simulink model "SingleTrack"  (R2019b)
settings: Solver=ode1  StartTime=0  StopTime=250  FixedStep=1.0000000000000000e-003  RelTol=1e-3
InitFcn:
  | sampleTime = str2double(get_param(bdroot, 'FixedStep'));
undefined symbols (not defined in the file or in its folder): AccPedalPos, BrakePedalPos, BrakeSwitch, DiscIntNeverNeededParam, DYNA4, EngSpd, IgnitionSwitch, InitialGear, InitialSpeed, IntendedEngTrq, LeftIndicator, MainBrakePress, MaxGear, MDL, MinGear, RefAcc, RefLane, RefLatPos, RefPath, RefPathCurv, RefSpd, RefSpdPreview, RefSpdRetrospect, RightIndicator, SteeringWheelAng, SteeringWheelTrq, UserDefinedRefValue, vm_const
libraries: UtilitiesLibrary x31, simulink x18, WheelSystemModules x13, LongitudinalControllerModules x13, LateralControllerModules x7, AnimationBusselectorModules x5, EnvironmentModules x5, BasicEngineControlModules x5, MiscellaneousControlModules x5, Animation3Modules x4, AuxiliariesModules x4, ReducedTireModules x4
(part 29 of 32)

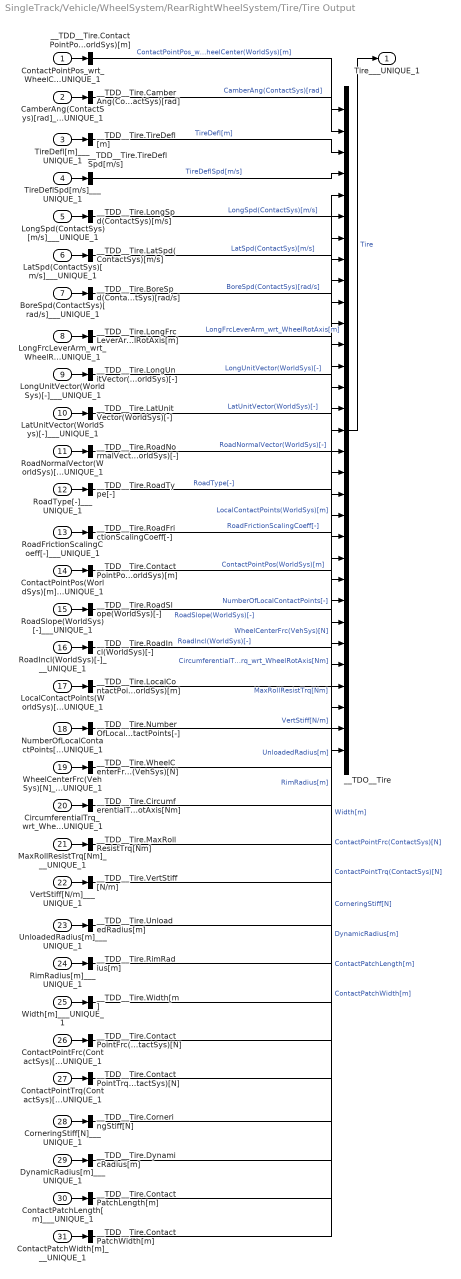
== system SingleTrack/Vehicle/WheelSystem/RearRightWheelSystem/Tire/Tire Output ==
  ContactPointPos_wrt_WheelCenter(WorldSys)[m]___UNIQUE_1 : Inport  Description=|  PortDimensions=[3]
      | <name>ContactPointPos_wrt_WheelCenter(WorldSys)[m]</name>
      | <comment></comment>
  CamberAng(ContactSys)[rad]___UNIQUE_1 : Inport  Description=|  Port=2  PortDimensions=[1]
      | <name>CamberAng(ContactSys)[rad]</name>
      | <comment></comment>
  TireDefl[m]___UNIQUE_1 : Inport  Description=|  Port=3  PortDimensions=[1]
      | <name>TireDefl[m]</name>
      | <comment></comment>
  TireDeflSpd[m/s]___UNIQUE_1 : Inport  Description=|  Port=4  PortDimensions=[1]
      | <name>TireDeflSpd[m/s]</name>
      | <comment></comment>
  LongSpd(ContactSys)[m/s]___UNIQUE_1 : Inport  Description=|  Port=5  PortDimensions=[1]
      | <name>LongSpd(ContactSys)[m/s]</name>
      | <comment></comment>
  LatSpd(ContactSys)[m/s]___UNIQUE_1 : Inport  Description=|  Port=6  PortDimensions=[1]
      | <name>LatSpd(ContactSys)[m/s]</name>
      | <comment></comment>
  BoreSpd(ContactSys)[rad/s]___UNIQUE_1 : Inport  Description=|  Port=7  PortDimensions=[1]
      | <name>BoreSpd(ContactSys)[rad/s]</name>
      | <comment></comment>
  LongFrcLeverArm_wrt_WheelRotAxis[m]___UNIQUE_1 : Inport  Description=|  Port=8  PortDimensions=[1]
      | <name>LongFrcLeverArm_wrt_WheelRotAxis[m]</name>
      | <comment></comment>
  LongUnitVector(WorldSys)[-]___UNIQUE_1 : Inport  Description=|  Port=9  PortDimensions=[3]
      | <name>LongUnitVector(WorldSys)[-]</name>
      | <comment></comment>
  LatUnitVector(WorldSys)[-]___UNIQUE_1 : Inport  Description=|  Port=10  PortDimensions=[3]
      | <name>LatUnitVector(WorldSys)[-]</name>
      | <comment></comment>
  RoadNormalVector(WorldSys)[-]___UNIQUE_1 : Inport  Description=|  Port=11  PortDimensions=[3]
      | <name>RoadNormalVector(WorldSys)[-]</name>
      | <comment></comment>
  RoadType[-]___UNIQUE_1 : Inport  Description=|  Port=12  PortDimensions=[1]
      | <name>RoadType[-]</name>
      | <comment></comment>
  RoadFrictionScalingCoeff[-]___UNIQUE_1 : Inport  Description=|  Port=13  PortDimensions=[1]
      | <name>RoadFrictionScalingCoeff[-]</name>
      | <comment></comment>
  ContactPointPos(WorldSys)[m]___UNIQUE_1 : Inport  Description=|  Port=14  PortDimensions=[3]
      | <name>ContactPointPos(WorldSys)[m]</name>
      | <comment></comment>
  RoadSlope(WorldSys)[-]___UNIQUE_1 : Inport  Description=|  Port=15  PortDimensions=[1]
      | <name>RoadSlope(WorldSys)[-]</name>
      | <comment></comment>
  RoadIncl(WorldSys)[-]___UNIQUE_1 : Inport  Description=|  Port=16  PortDimensions=[1]
      | <name>RoadIncl(WorldSys)[-]</name>
      | <comment></comment>
  LocalContactPoints(WorldSys)[m]___UNIQUE_1 : Inport  Description=|  Port=17  PortDimensions=[12]
      | <name>LocalContactPoints(WorldSys)[m]</name>
      | <comment></comment>
  NumberOfLocalContactPoints[-]___UNIQUE_1 : Inport  Description=|  Port=18  PortDimensions=[1]
      | <name>NumberOfLocalContactPoints[-]</name>
      | <comment></comment>
  WheelCenterFrc(VehSys)[N]___UNIQUE_1 : Inport  Description=|  Port=19  PortDimensions=[3]
      | <name>WheelCenterFrc(VehSys)[N]</name>
      | <comment></comment>
  CircumferentialTrq_wrt_WheelRotAxis[Nm]___UNIQUE_1 : Inport  Description=|  Port=20  PortDimensions=[1]
      | <name>CircumferentialTrq_wrt_WheelRotAxis[Nm]</name>
      | <comment></comment>
  MaxRollResistTrq[Nm]___UNIQUE_1 : Inport  Description=|  Port=21  PortDimensions=[1]
      | <name>MaxRollResistTrq[Nm]</name>
      | <comment></comment>
  VertStiff[N/m]___UNIQUE_1 : Inport  Description=|  Port=22  PortDimensions=[1]
      | <name>VertStiff[N/m]</name>
      | <comment></comment>
  UnloadedRadius[m]___UNIQUE_1 : Inport  Description=|  Port=23  PortDimensions=[1]
      | <name>UnloadedRadius[m]</name>
      | <comment></comment>
  RimRadius[m]___UNIQUE_1 : Inport  Description=|  Port=24  PortDimensions=[1]
      | <name>RimRadius[m]</name>
      | <comment></comment>
  Width[m]___UNIQUE_1 : Inport  Description=|  Port=25  PortDimensions=[1]
      | <name>Width[m]</name>
      | <comment></comment>
  ContactPointFrc(ContactSys)[N]___UNIQUE_1 : Inport  Description=|  Port=26  PortDimensions=[3]
      | <name>ContactPointFrc(ContactSys)[N]</name>
      | <comment></comment>
  ContactPointTrq(ContactSys)[N]___UNIQUE_1 : Inport  Description=|  Port=27  PortDimensions=[3]
      | <name>ContactPointTrq(ContactSys)[N]</name>
      | <comment></comment>
  CorneringStiff[N]___UNIQUE_1 : Inport  Description=|  Port=28  PortDimensions=[1]
      | <name>CorneringStiff[N]</name>
      | <comment></comment>
  DynamicRadius[m]___UNIQUE_1 : Inport  Description=|  Port=29  PortDimensions=[1]
      | <name>DynamicRadius[m]</name>
      | <comment></comment>
  ContactPatchLength[m]___UNIQUE_1 : Inport  Description=|  Port=30  PortDimensions=[1]
      | <name>ContactPatchLength[m]</name>
      | <comment></comment>
  ContactPatchWidth[m]___UNIQUE_1 : Inport  Description=|  Port=31  PortDimensions=[1]
      | <name>ContactPatchWidth[m]</name>
      | <comment></comment>
  __TDD__Tire.BoreSpd(ContactSys)[rad/s] : Demux  Outputs=[1]
  __TDD__Tire.CamberAng(ContactSys)[rad] : Demux  Outputs=[1]
  __TDD__Tire.CircumferentialTrq_wrt_WheelRotAxis[Nm] : Demux  Outputs=[1]
  __TDD__Tire.ContactPatchLength[m] : Demux  Outputs=[1]
  __TDD__Tire.ContactPatchWidth[m] : Demux  Outputs=[1]
  __TDD__Tire.ContactPointFrc(ContactSys)[N] : Demux  Outputs=[3]
  __TDD__Tire.ContactPointPos(WorldSys)[m] : Demux  Outputs=[3]
  __TDD__Tire.ContactPointPos_wrt_WheelCenter(WorldSys)[m] : Demux  Outputs=[3]
  __TDD__Tire.ContactPointTrq(ContactSys)[N] : Demux  Outputs=[3]
  __TDD__Tire.CorneringStiff[N] : Demux  Outputs=[1]
  __TDD__Tire.DynamicRadius[m] : Demux  Outputs=[1]
  __TDD__Tire.LatSpd(ContactSys)[m/s] : Demux  Outputs=[1]
  __TDD__Tire.LatUnitVector(WorldSys)[-] : Demux  Outputs=[3]
  __TDD__Tire.LocalContactPoints(WorldSys)[m] : Demux  Outputs=[12]
  __TDD__Tire.LongFrcLeverArm_wrt_WheelRotAxis[m] : Demux  Outputs=[1]
  __TDD__Tire.LongSpd(ContactSys)[m/s] : Demux  Outputs=[1]
  __TDD__Tire.LongUnitVector(WorldSys)[-] : Demux  Outputs=[3]
  __TDD__Tire.MaxRollResistTrq[Nm] : Demux  Outputs=[1]
  __TDD__Tire.NumberOfLocalContactPoints[-] : Demux  Outputs=[1]
  __TDD__Tire.RimRadius[m] : Demux  Outputs=[1]
  __TDD__Tire.RoadFrictionScalingCoeff[-] : Demux  Outputs=[1]
  __TDD__Tire.RoadIncl(WorldSys)[-] : Demux  Outputs=[1]
  __TDD__Tire.RoadNormalVector(WorldSys)[-] : Demux  Outputs=[3]
  __TDD__Tire.RoadSlope(WorldSys)[-] : Demux  Outputs=[1]
  __TDD__Tire.RoadType[-] : Demux  Outputs=[1]
  __TDD__Tire.TireDeflSpd[m/s] : Demux  Outputs=[1]
  __TDD__Tire.TireDefl[m] : Demux  Outputs=[1]
  __TDD__Tire.UnloadedRadius[m] : Demux  Outputs=[1]
  __TDD__Tire.VertStiff[N/m] : Demux  Outputs=[1]
  __TDD__Tire.WheelCenterFrc(VehSys)[N] : Demux  Outputs=[3]
  __TDD__Tire.Width[m] : Demux  Outputs=[1]
  __TDO__Tire : BusCreator  Inputs=31
  Tire___UNIQUE_1 : Outport  Description=|  PortDimensions=[58]  VectorParamsAs1DForOutWhenUnconnected=off
      | <name>ContactPointPos_wrt_WheelCenter(WorldSys)[m]</name>
      | <comment></comment>
  wires:
  __TDO__Tire/1 -> Tire___UNIQUE_1/1  "Tire"
  __TDD__Tire.ContactPatchWidth[m]/1 -> __TDO__Tire/31  "ContactPatchWidth[m]"
  ContactPatchWidth[m]___UNIQUE_1/1 -> __TDD__Tire.ContactPatchWidth[m]/1
  __TDD__Tire.ContactPatchLength[m]/1 -> __TDO__Tire/30  "ContactPatchLength[m]"
  ContactPatchLength[m]___UNIQUE_1/1 -> __TDD__Tire.ContactPatchLength[m]/1
  __TDD__Tire.DynamicRadius[m]/1 -> __TDO__Tire/29  "DynamicRadius[m]"
  DynamicRadius[m]___UNIQUE_1/1 -> __TDD__Tire.DynamicRadius[m]/1
  __TDD__Tire.CorneringStiff[N]/1 -> __TDO__Tire/28  "CorneringStiff[N]"
  CorneringStiff[N]___UNIQUE_1/1 -> __TDD__Tire.CorneringStiff[N]/1
  __TDD__Tire.ContactPointTrq(ContactSys)[N]/1 -> __TDO__Tire/27  "ContactPointTrq(ContactSys)[N]"
  ContactPointTrq(ContactSys)[N]___UNIQUE_1/1 -> __TDD__Tire.ContactPointTrq(ContactSys)[N]/1
  __TDD__Tire.ContactPointFrc(ContactSys)[N]/1 -> __TDO__Tire/26  "ContactPointFrc(ContactSys)[N]"
  ContactPointFrc(ContactSys)[N]___UNIQUE_1/1 -> __TDD__Tire.ContactPointFrc(ContactSys)[N]/1
  __TDD__Tire.Width[m]/1 -> __TDO__Tire/25  "Width[m]"
  Width[m]___UNIQUE_1/1 -> __TDD__Tire.Width[m]/1
  __TDD__Tire.RimRadius[m]/1 -> __TDO__Tire/24  "RimRadius[m]"
  RimRadius[m]___UNIQUE_1/1 -> __TDD__Tire.RimRadius[m]/1
  __TDD__Tire.UnloadedRadius[m]/1 -> __TDO__Tire/23  "UnloadedRadius[m]"
  UnloadedRadius[m]___UNIQUE_1/1 -> __TDD__Tire.UnloadedRadius[m]/1
  __TDD__Tire.VertStiff[N/m]/1 -> __TDO__Tire/22  "VertStiff[N/m]"
  VertStiff[N/m]___UNIQUE_1/1 -> __TDD__Tire.VertStiff[N/m]/1
  __TDD__Tire.MaxRollResistTrq[Nm]/1 -> __TDO__Tire/21  "MaxRollResistTrq[Nm]"
  MaxRollResistTrq[Nm]___UNIQUE_1/1 -> __TDD__Tire.MaxRollResistTrq[Nm]/1
  __TDD__Tire.CircumferentialTrq_wrt_WheelRotAxis[Nm]/1 -> __TDO__Tire/20  "CircumferentialTrq_wrt_WheelRotAxis[Nm]"
  CircumferentialTrq_wrt_WheelRotAxis[Nm]___UNIQUE_1/1 -> __TDD__Tire.CircumferentialTrq_wrt_WheelRotAxis[Nm]/1
  __TDD__Tire.WheelCenterFrc(VehSys)[N]/1 -> __TDO__Tire/19  "WheelCenterFrc(VehSys)[N]"
  WheelCenterFrc(VehSys)[N]___UNIQUE_1/1 -> __TDD__Tire.WheelCenterFrc(VehSys)[N]/1
  __TDD__Tire.NumberOfLocalContactPoints[-]/1 -> __TDO__Tire/18  "NumberOfLocalContactPoints[-]"
  NumberOfLocalContactPoints[-]___UNIQUE_1/1 -> __TDD__Tire.NumberOfLocalContactPoints[-]/1
  __TDD__Tire.LocalContactPoints(WorldSys)[m]/1 -> __TDO__Tire/17  "LocalContactPoints(WorldSys)[m]"
  LocalContactPoints(WorldSys)[m]___UNIQUE_1/1 -> __TDD__Tire.LocalContactPoints(WorldSys)[m]/1
  __TDD__Tire.RoadIncl(WorldSys)[-]/1 -> __TDO__Tire/16  "RoadIncl(WorldSys)[-]"
  RoadIncl(WorldSys)[-]___UNIQUE_1/1 -> __TDD__Tire.RoadIncl(WorldSys)[-]/1
  __TDD__Tire.RoadSlope(WorldSys)[-]/1 -> __TDO__Tire/15  "RoadSlope(WorldSys)[-]"
  RoadSlope(WorldSys)[-]___UNIQUE_1/1 -> __TDD__Tire.RoadSlope(WorldSys)[-]/1
  __TDD__Tire.ContactPointPos(WorldSys)[m]/1 -> __TDO__Tire/14  "ContactPointPos(WorldSys)[m]"
  ContactPointPos(WorldSys)[m]___UNIQUE_1/1 -> __TDD__Tire.ContactPointPos(WorldSys)[m]/1
  __TDD__Tire.RoadFrictionScalingCoeff[-]/1 -> __TDO__Tire/13  "RoadFrictionScalingCoeff[-]"
  RoadFrictionScalingCoeff[-]___UNIQUE_1/1 -> __TDD__Tire.RoadFrictionScalingCoeff[-]/1
  __TDD__Tire.RoadType[-]/1 -> __TDO__Tire/12  "RoadType[-]"
  RoadType[-]___UNIQUE_1/1 -> __TDD__Tire.RoadType[-]/1
  __TDD__Tire.RoadNormalVector(WorldSys)[-]/1 -> __TDO__Tire/11  "RoadNormalVector(WorldSys)[-]"
  RoadNormalVector(WorldSys)[-]___UNIQUE_1/1 -> __TDD__Tire.RoadNormalVector(WorldSys)[-]/1
  __TDD__Tire.LatUnitVector(WorldSys)[-]/1 -> __TDO__Tire/10  "LatUnitVector(WorldSys)[-]"
  LatUnitVector(WorldSys)[-]___UNIQUE_1/1 -> __TDD__Tire.LatUnitVector(WorldSys)[-]/1
  __TDD__Tire.LongUnitVector(WorldSys)[-]/1 -> __TDO__Tire/9  "LongUnitVector(WorldSys)[-]"
  LongUnitVector(WorldSys)[-]___UNIQUE_1/1 -> __TDD__Tire.LongUnitVector(WorldSys)[-]/1
  __TDD__Tire.LongFrcLeverArm_wrt_WheelRotAxis[m]/1 -> __TDO__Tire/8  "LongFrcLeverArm_wrt_WheelRotAxis[m]"
  LongFrcLeverArm_wrt_WheelRotAxis[m]___UNIQUE_1/1 -> __TDD__Tire.LongFrcLeverArm_wrt_WheelRotAxis[m]/1
  __TDD__Tire.BoreSpd(ContactSys)[rad/s]/1 -> __TDO__Tire/7  "BoreSpd(ContactSys)[rad/s]"
  BoreSpd(ContactSys)[rad/s]___UNIQUE_1/1 -> __TDD__Tire.BoreSpd(ContactSys)[rad/s]/1
  __TDD__Tire.LatSpd(ContactSys)[m/s]/1 -> __TDO__Tire/6  "LatSpd(ContactSys)[m/s]"
  LatSpd(ContactSys)[m/s]___UNIQUE_1/1 -> __TDD__Tire.LatSpd(ContactSys)[m/s]/1
  __TDD__Tire.LongSpd(ContactSys)[m/s]/1 -> __TDO__Tire/5  "LongSpd(ContactSys)[m/s]"
  LongSpd(ContactSys)[m/s]___UNIQUE_1/1 -> __TDD__Tire.LongSpd(ContactSys)[m/s]/1
  __TDD__Tire.TireDeflSpd[m/s]/1 -> __TDO__Tire/4  "TireDeflSpd[m/s]"
  TireDeflSpd[m/s]___UNIQUE_1/1 -> __TDD__Tire.TireDeflSpd[m/s]/1
  __TDD__Tire.TireDefl[m]/1 -> __TDO__Tire/3  "TireDefl[m]"
  TireDefl[m]___UNIQUE_1/1 -> __TDD__Tire.TireDefl[m]/1
  __TDD__Tire.CamberAng(ContactSys)[rad]/1 -> __TDO__Tire/2  "CamberAng(ContactSys)[rad]"
  CamberAng(ContactSys)[rad]___UNIQUE_1/1 -> __TDD__Tire.CamberAng(ContactSys)[rad]/1
  __TDD__Tire.ContactPointPos_wrt_WheelCenter(WorldSys)[m]/1 -> __TDO__Tire/1  "ContactPointPos_wrt_WheelCenter(WorldSys)[m]"
  ContactPointPos_wrt_WheelCenter(WorldSys)[m]___UNIQUE_1/1 -> __TDD__Tire.ContactPointPos_wrt_WheelCenter(WorldSys)[m]/1

== system SingleTrack/Vehicle/WheelSystem/WheelSystemOutputs/WheelRear2//3Output/WheelSystemOutput ==
  __SEL__WheelSystem.InnerTire.ContactPointFrc(ContactSys)[N] : Selector  InputPortWidth=1  IndexOptions=Index vector (dialog)  Indices=ones(3, 1)  OutputSizes=1
  __SEL__WheelSystem.InnerTire.ContactPointPos(WorldSys)[m] : Selector  InputPortWidth=1  IndexOptions=Index vector (dialog)  Indices=ones(3, 1)  OutputSizes=1
  __SEL__WheelSystem.Tire.ContactPointFrc(ContactSys)[N] : Selector  InputPortWidth=1  IndexOptions=Index vector (dialog)  Indices=ones(3, 1)  OutputSizes=1
  __SEL__WheelSystem.Tire.ContactPointPos(WorldSys)[m] : Selector  InputPortWidth=1  IndexOptions=Index vector (dialog)  Indices=ones(3, 1)  OutputSizes=1
  __SRC__WheelSystem.InnerTire.ContactPointFrc(ContactSys)[N] : Constant  Value=0.0  OutDataTypeStr=Inherit: Inherit via back propagation
  __SRC__WheelSystem.InnerTire.ContactPointPos(WorldSys)[m] : Constant  Value=0.0  OutDataTypeStr=Inherit: Inherit via back propagation
  __SRC__WheelSystem.InnerTire.MaxRollResistTrq[Nm] : Constant  Value=0.0  OutDataTypeStr=Inherit: Inherit via back propagation
  __SRC__WheelSystem.Tire.ContactPointFrc(ContactSys)[N] : Constant  Value=0.0  OutDataTypeStr=Inherit: Inherit via back propagation
  __SRC__WheelSystem.Tire.ContactPointPos(WorldSys)[m] : Constant  Value=0.0  OutDataTypeStr=Inherit: Inherit via back propagation
  __SRC__WheelSystem.Tire.MaxRollResistTrq[Nm] : Constant  Value=0.0  OutDataTypeStr=Inherit: Inherit via back propagation
  __SRC__WheelSystem.Wheel.RotAcc[rad/s**2] : Constant  Value=0.0  OutDataTypeStr=Inherit: Inherit via back propagation
  __SRC__WheelSystem.Wheel.RotAng[rad] : Constant  Value=0.0  OutDataTypeStr=Inherit: Inherit via back propagation
  __SRC__WheelSystem.Wheel.RotAxisInrt[kg*m**2] : Constant  Value=0.0  OutDataTypeStr=Inherit: Inherit via back propagation
  __SRC__WheelSystem.Wheel.RotSpd[rad/s] : Constant  Value=0.0  OutDataTypeStr=Inherit: Inherit via back propagation
  __TDO__WheelSystem : BusCreator  Inputs=3
  __TDO__WheelSystem.InnerTire : BusCreator  Inputs=3
  __TDO__WheelSystem.Tire : BusCreator  Inputs=3
  __TDO__WheelSystem.Wheel : BusCreator  Inputs=4
  WheelSystem___UNIQUE_1 : Outport  Description=|  PortDimensions=[18]  VectorParamsAs1DForOutWhenUnconnected=off
      | <name></name>
      | <comment></comment>
  wires:
  __TDO__WheelSystem/1 -> WheelSystem___UNIQUE_1/1  "WheelSystem"
  __SEL__WheelSystem.InnerTire.ContactPointFrc(ContactSys)[N]/1 -> __TDO__WheelSystem.InnerTire/3  "ContactPointFrc(ContactSys)[N]"
  __SEL__WheelSystem.InnerTire.ContactPointPos(WorldSys)[m]/1 -> __TDO__WheelSystem.InnerTire/2  "ContactPointPos(WorldSys)[m]"
  __SEL__WheelSystem.Tire.ContactPointFrc(ContactSys)[N]/1 -> __TDO__WheelSystem.Tire/3  "ContactPointFrc(ContactSys)[N]"
  __SEL__WheelSystem.Tire.ContactPointPos(WorldSys)[m]/1 -> __TDO__WheelSystem.Tire/2  "ContactPointPos(WorldSys)[m]"
  __SRC__WheelSystem.Wheel.RotAng[rad]/1 -> __TDO__WheelSystem.Wheel/4  "RotAng[rad]"
  __TDO__WheelSystem.InnerTire/1 -> __TDO__WheelSystem/3  "InnerTire"
  __SRC__WheelSystem.InnerTire.MaxRollResistTrq[Nm]/1 -> __TDO__WheelSystem.InnerTire/1  "MaxRollResistTrq[Nm]"
  __TDO__WheelSystem.Tire/1 -> __TDO__WheelSystem/2  "Tire"
  __SRC__WheelSystem.Tire.MaxRollResistTrq[Nm]/1 -> __TDO__WheelSystem.Tire/1  "MaxRollResistTrq[Nm]"
  __SRC__WheelSystem.Wheel.RotAxisInrt[kg*m**2]/1 -> __TDO__WheelSystem.Wheel/3  "RotAxisInrt[kg*m**2]"
  __SRC__WheelSystem.Wheel.RotAcc[rad/s**2]/1 -> __TDO__WheelSystem.Wheel/2  "RotAcc[rad/s**2]"
  __TDO__WheelSystem.Wheel/1 -> __TDO__WheelSystem/1  "Wheel"
  __SRC__WheelSystem.Wheel.RotSpd[rad/s]/1 -> __TDO__WheelSystem.Wheel/1  "RotSpd[rad/s]"
  __SRC__WheelSystem.InnerTire.ContactPointFrc(ContactSys)[N]/1 -> __SEL__WheelSystem.InnerTire.ContactPointFrc(ContactSys)[N]/1
  __SRC__WheelSystem.InnerTire.ContactPointPos(WorldSys)[m]/1 -> __SEL__WheelSystem.InnerTire.ContactPointPos(WorldSys)[m]/1
  __SRC__WheelSystem.Tire.ContactPointFrc(ContactSys)[N]/1 -> __SEL__WheelSystem.Tire.ContactPointFrc(ContactSys)[N]/1
  __SRC__WheelSystem.Tire.ContactPointPos(WorldSys)[m]/1 -> __SEL__WheelSystem.Tire.ContactPointPos(WorldSys)[m]/1

== system SingleTrack/VehicleControl/LateralControl/Disabled LateralControl/ControlSystems/Control Systems Parameters ==
  CurvatureControl : Subsystem
      settings: CopyFcn=DYNA4.Internal.ModelCallbacks.Modules.UpdateMaskParameters(gcb);  NameChangeFcn=DYNA4.Internal.ModelCallbacks.Modules.UpdateMaskParameters(gcb);
  PathControl : Subsystem
      settings: CopyFcn=DYNA4.Internal.ModelCallbacks.Modules.UpdateMaskParameters(gcb);  NameChangeFcn=DYNA4.Internal.ModelCallbacks.Modules.UpdateMaskParameters(gcb);

== system SingleTrack/VehicleControl/LateralControl/Disabled LateralControl/ControlSystems/DynaSystemInfo ==

== system SingleTrack/VehicleControl/LateralControl/Disabled LateralControl/ControlSystems/Lateral Controller ==
  User-Defined Control : Subsystem  TreatAsAtomicUnit=on

== system SingleTrack/VehicleControl/LateralControl/Disabled LateralControl/ControlSystems/LateralControlOutput ==
  __SRC__LateralControl.LateralPhase : Constant  Value=0.0  OutDataTypeStr=Inherit: Inherit via back propagation
  __SRC__LateralControl.LeftIndicator : Constant  Value=0.0  OutDataTypeStr=Inherit: Inherit via back propagation
  __SRC__LateralControl.RightIndicator : Constant  Value=0.0  OutDataTypeStr=Inherit: Inherit via back propagation
  __SRC__LateralControl.SteeringWheelAng : Constant  Value=0.0  OutDataTypeStr=Inherit: Inherit via back propagation
  __SRC__LateralControl.SteeringWheelInputSwitch : Constant  Value=0.0  OutDataTypeStr=Inherit: Inherit via back propagation
  __SRC__LateralControl.SteeringWheelTrq : Constant  Value=0.0  OutDataTypeStr=Inherit: Inherit via back propagation
  __SRC__LateralControl.UserDefined1 : Constant  Value=0.0  OutDataTypeStr=Inherit: Inherit via back propagation
  __SRC__LateralControl.UserDefined2 : Constant  Value=0.0  OutDataTypeStr=Inherit: Inherit via back propagation
  __SRC__LateralControl.UserDefinedRefValue : Constant  Value=0.0  OutDataTypeStr=Inherit: Inherit via back propagation
  __TDO__LateralControl : BusCreator  Inputs=9
  LateralControl___UNIQUE_1 : Outport  Description=|  PortDimensions=[9]  VectorParamsAs1DForOutWhenUnconnected=off
      | <name>SteeringWheelAng</name>
      | <comment>Steering wheel angle</comment>
  wires:
  __TDO__LateralControl/1 -> LateralControl___UNIQUE_1/1  "LateralControl"
  __SRC__LateralControl.UserDefined2/1 -> __TDO__LateralControl/9  "UserDefined2[-]"
  __SRC__LateralControl.UserDefined1/1 -> __TDO__LateralControl/8  "UserDefined1[-]"
  __SRC__LateralControl.LateralPhase/1 -> __TDO__LateralControl/7  "LateralPhase[-]"
  __SRC__LateralControl.RightIndicator/1 -> __TDO__LateralControl/6  "RightIndicator[0;1]"
  __SRC__LateralControl.LeftIndicator/1 -> __TDO__LateralControl/5  "LeftIndicator[0;1]"
  __SRC__LateralControl.UserDefinedRefValue/1 -> __TDO__LateralControl/4  "UserDefinedRefValue[-]"
  __SRC__LateralControl.SteeringWheelInputSwitch/1 -> __TDO__LateralControl/3  "SteeringWheelInputSwitch[-]"
  __SRC__LateralControl.SteeringWheelTrq/1 -> __TDO__LateralControl/2  "SteeringWheelTrq[Nm]"
  __SRC__LateralControl.SteeringWheelAng/1 -> __TDO__LateralControl/1  "SteeringWheelAng[rad]"

== system SingleTrack/VehicleControl/LateralControl/Disabled LateralControl/ControlSystemsPreprocessor/Maneuver ==
  DynaModuleInfo : Subsystem  Tag=DynaModuleInfo
      mask init:
      | data = get_param(gcb, 'UserData');
      mask Display: disp(['Type = ', data.type, '\nName = ', char(data.name)]);

== system SingleTrack/VehicleControl/LateralControl/Enabled LateralControl/ControlSystems/Control Systems Parameters ==
  note: TASK_LAT_STEERING_WHEEL_ANG = 1;
      | 	TASK_LAT_STEERING_WHEEL_TORQUE = 2;
      | 	TASK_LAT_PATH_CONTROL = 3;
      | 	TASK_LAT_CURVATURE_CONTROL = 4;
      | 	TASK_LAT_USER_DEFINED = 5;
  TaskIdentifier : Inport
  CtrlSystemsAbscissae : Inport  Port=2
  Bus Selector : BusSelector  OutputSignals=Task
  CurvatureControl : LateralControllerModules/DataContainerCurvatureControl  DATA_NODE=MDL.VehicleControl.LateralControl.ControlSystems.CurvatureControl  PreviewDist=MDL.VehicleControl.LateralControl.ControlSystems.CurvatureControl.PreviewDist  PreviewTime=MDL.VehicleControl.LateralControl.ControlSystems.CurvatureControl.PreviewTime  TargetAimDist=MDL.VehicleControl.LateralControl.ControlSystems.CurvatureControl.TargetAimDist  MaxLeftSteeringRate=MDL.VehicleControl.LateralControl.ControlSystems.CurvatureControl.MaxLeftSteeringRate  MaxRightSteeringRate=MDL.VehicleControl.LateralControl.ControlSystems.CurvatureControl.MaxRightSteeringRate  SteeringAngSmoothTimeConst=MDL.VehicleControl.LateralControl.ControlSystems.CurvatureControl.SteeringAngSmoothTimeConst  LatCtrlGain=MDL.VehicleControl.LateralControl.ControlSystems.CurvatureControl.LatCtrlGain  ControllerDeviationScaling=MDL.VehicleControl.LateralControl.ControlSystems.CurvatureControl.ControllerDeviationScaling  FrontAxleLatStiff=MDL.VehicleControl.LateralControl.ControlSystems.CurvatureControl.FrontAxleLatStiff  RearAxleLatStiff=MDL.VehicleControl.LateralControl.ControlSystems.CurvatureControl.RearAxleLatStiff  RearTiresLatFrcSmoothTimeConst=MDL.VehicleControl.LateralControl.ControlSystems.CurvatureControl.RearTiresLatFrcSmoothTimeConst  RearTiresLatFrcSwitch=MDL.VehicleControl.LateralControl.ControlSystems.CurvatureControl.RearTiresLatFrcSwitch  RearTiresLatFrcScaling=MDL.VehicleControl.LateralControl.ControlSystems.CurvatureControl.RearTiresLatFrcScaling  SmoothingInterval=MDL.VehicleControl.LateralControl.ControlSystems.CurvatureControl.SmoothingInterval  Preview=MDL.VehicleControl.LateralControl.ControlSystems.CurvatureControl.Preview  DrivingSkill=MDL.VehicleControl.LateralControl.ControlSystems.CurvatureControl.DrivingSkill  Smoothness=MDL.VehicleControl.LateralControl.ControlSystems.CurvatureControl.Smoothness
  Merge : Merge
  PathControl : LateralControllerModules/DataContainerPathControl  DATA_NODE=MDL.VehicleControl.LateralControl.ControlSystems.PathControl  PreviewDist=MDL.VehicleControl.LateralControl.ControlSystems.PathControl.PreviewDist  PreviewTime=MDL.VehicleControl.LateralControl.ControlSystems.PathControl.PreviewTime  TargetAimDist=MDL.VehicleControl.LateralControl.ControlSystems.PathControl.TargetAimDist  MaxLeftSteeringRate=MDL.VehicleControl.LateralControl.ControlSystems.PathControl.MaxLeftSteeringRate  MaxRightSteeringRate=MDL.VehicleControl.LateralControl.ControlSystems.PathControl.MaxRightSteeringRate  SteeringAngSmoothTimeConst=MDL.VehicleControl.LateralControl.ControlSystems.PathControl.SteeringAngSmoothTimeConst  LatCtrlGain=MDL.VehicleControl.LateralControl.ControlSystems.PathControl.LatCtrlGain  ControllerDeviationScaling=MDL.VehicleControl.LateralControl.ControlSystems.PathControl.ControllerDeviationScaling  FrontAxleLatStiff=MDL.VehicleControl.LateralControl.ControlSystems.PathControl.FrontAxleLatStiff  RearAxleLatStiff=MDL.VehicleControl.LateralControl.ControlSystems.PathControl.RearAxleLatStiff  RearTiresLatFrcSmoothTimeConst=MDL.VehicleControl.LateralControl.ControlSystems.PathControl.RearTiresLatFrcSmoothTimeConst  RearTiresLatFrcSwitch=MDL.VehicleControl.LateralControl.ControlSystems.PathControl.RearTiresLatFrcSwitch  RearTiresLatFrcScaling=MDL.VehicleControl.LateralControl.ControlSystems.PathControl.RearTiresLatFrcScaling  LaneChangeDurationTime=MDL.VehicleControl.LateralControl.ControlSystems.PathControl.LaneChangeDurationTime  LaneChangeDurationDist=MDL.VehicleControl.LateralControl.ControlSystems.PathControl.LaneChangeDurationDist  SmoothingInterval=MDL.VehicleControl.LateralControl.ControlSystems.PathControl.SmoothingInterval  Preview=MDL.VehicleControl.LateralControl.ControlSystems.PathControl.Preview  DrivingSkill=MDL.VehicleControl.LateralControl.ControlSystems.PathControl.DrivingSkill  Smoothness=MDL.VehicleControl.LateralControl.ControlSystems.PathControl.Smoothness
  Switch Case : SwitchCase  CaseConditions={vm_const('TASK_LAT_PATH_CONTROL'), vm_const('TASK_LAT_CURVATURE_CONTROL')}  ShowDefaultCase=off
  ControllerParameters : Outport  VectorParamsAs1DForOutWhenUnconnected=off
  wires:
  Switch Case/2 -> CurvatureControl/Action
  Switch Case/1 -> PathControl/Action
  CtrlSystemsAbscissae/1 -> CurvatureControl/1, PathControl/1
  Merge/1 -> ControllerParameters/1
  CurvatureControl/1 -> Merge/2
  PathControl/1 -> Merge/1
  TaskIdentifier/1 -> Bus Selector/1
  Bus Selector/1 -> Switch Case/1  "<Task>"

== system SingleTrack/VehicleControl/LateralControl/Enabled LateralControl/ControlSystems/DynaSystemInfo ==

== system SingleTrack/VehicleControl/LateralControl/Enabled LateralControl/ControlSystems/Lateral Controller ==
  note: TASK_LAT_STEERING_WHEEL_ANG = 1;
      | 	TASK_LAT_STEERING_WHEEL_TORQUE = 2;
      | 	TASK_LAT_PATH_CONTROL = 3;
      | 	TASK_LAT_CURVATURE_CONTROL = 4;
      | 	TASK_LAT_USER_DEFINED = 5;
  TaskIdentifiers : Inport
  SourceIdentifiers : Inport  Port=2
  ControlInputs : Inport  Port=3
  ControllerParameters : Inport  Port=4
  VehicleInfo : Inport  Port=5
  Bus Selector : BusSelector  OutputSignals=Task,Subtask
  Initialization : Subsystem
  Merge : Merge  Inputs=5
  Path and Curvature Control : Subsystem  TreatAsAtomicUnit=on
  Steering Wheel Angle Input : Subsystem  TreatAsAtomicUnit=on
  Steering Wheel Torque Input : Subsystem  TreatAsAtomicUnit=on
  Switch Case : SwitchCase  CaseConditions={vm_const('TASK_LAT_STEERING_WHEEL_ANG'), vm_const('TASK_LAT_STEERING_WHEEL_TORQUE'), [vm_const('TASK_LAT_PATH_CONTROL'),vm_const('TASK_LAT_CURVATURE_CONTROL')], vm_const('TASK_LAT_USER_DEFINED')}
  User-Defined Control : Subsystem  TreatAsAtomicUnit=on
  SteeringWheelDemands : Outport  VectorParamsAs1DForOutWhenUnconnected=off
  UserDefinedRefValue[-] : Outport  Port=2  PortDimensions=1  VectorParamsAs1DForOutWhenUnconnected=off
  wires:
  Steering Wheel Torque Input/1(SteeringWheelDemands) -> Merge/2
  Switch Case/2 -> Steering Wheel Torque Input/Action
  User-Defined Control/1(SteeringWheelDemands) -> Merge/4
  Path and Curvature Control/1(SteeringWheelDemands) -> Merge/3
  Initialization/1(SteeringWheelDemands) -> Merge/5
  Switch Case/3 -> Path and Curvature Control/Action
  Switch Case/4 -> User-Defined Control/Action
  Switch Case/1 -> Steering Wheel Angle Input/Action
  Switch Case/5 -> Initialization/Action
  User-Defined Control/2(UserDefinedRefValue[-]) -> UserDefinedRefValue[-]/1
  SourceIdentifiers/1 -> User-Defined Control/3(SourceIdentifiers)
  ControlInputs/1 -> Steering Wheel Angle Input/1(ControlInputs), Steering Wheel Torque Input/1(ControlInputs), Path and Curvature Control/1(ControlInputs), User-Defined Control/1(ControlInputs)
  ControllerParameters/1 -> Path and Curvature Control/2(ControllerParameters)
  VehicleInfo/1 -> Path and Curvature Control/3(VehicleInfo), User-Defined Control/2(VehicleInfo), Steering Wheel Angle Input/2(VehicleInfo), Steering Wheel Torque Input/2(VehicleInfo)
  Merge/1 -> SteeringWheelDemands/1
  Steering Wheel Angle Input/1(SteeringWheelDemands) -> Merge/1
  TaskIdentifiers/1 -> Bus Selector/1
  Bus Selector/1 -> Switch Case/1  "<Task>"
  Bus Selector/2 -> User-Defined Control/4(SubtaskIdentifiers)  "<Subtask>"

== system SingleTrack/VehicleControl/LateralControl/Enabled LateralControl/ControlSystems/LateralControlOutput ==
  SteeringWheelAng[rad]___UNIQUE_1 : Inport  Description=|  PortDimensions=[1]
      | <name>SteeringWheelAng[rad]</name>
      | <comment>Steering wheel angle</comment>
  SteeringWheelTrq[Nm]___UNIQUE_1 : Inport  Description=|  Port=2  PortDimensions=[1]
      | <name>SteeringWheelTrq[Nm]</name>
      | <comment>Steering wheel torque</comment>
  SteeringWheelInputSwitch[-]___UNIQUE_1 : Inport  Description=|  Port=3  PortDimensions=[1]
      | <name>SteeringWheelInputSwitch[-]</name>
      | <comment>Steering wheel input switch (0: angle, 1: torque)</comment>
  UserDefinedRefValue[-]___UNIQUE_1 : Inport  Description=|  Port=4  PortDimensions=[1]
      | <name>UserDefinedRefValue[-]</name>
      | <comment>User-defined reference value</comment>
  LeftIndicator[0;1]___UNIQUE_1 : Inport  Description=|  Port=5  PortDimensions=[1]
      | <name>LeftIndicator[0;1]</name>
      | <comment>Left indicator state</comment>
  RightIndicator[0;1]___UNIQUE_1 : Inport  Description=|  Port=6  PortDimensions=[1]
      | <name>RightIndicator[0;1]</name>
      | <comment>Right indicator state</comment>
  LateralPhase[-]___UNIQUE_1 : Inport  Description=|  Port=7  PortDimensions=[1]
      | <name>LateralPhase[-]</name>
      | <comment>Lateral phase number</comment>
  UserDefined1[-]___UNIQUE_1 : Inport  Description=|  Port=8  PortDimensions=[1]
      | <name>UserDefined.UserDefined1[-]</name>
      | <comment>User-defined additional input 1 (can be edited by the user)</comment>
  UserDefined2[-]___UNIQUE_1 : Inport  Description=|  Port=9  PortDimensions=[1]
      | <name>UserDefined.UserDefined2[-]</name>
      | <comment>User-defined additional input 2 (can be edited by the user)</comment>
  __TDD__LateralControl.LateralPhase[-] : Demux  Outputs=[1]
  __TDD__LateralControl.LeftIndicator[0;1] : Demux  Outputs=[1]
  __TDD__LateralControl.RightIndicator[0;1] : Demux  Outputs=[1]
  __TDD__LateralControl.SteeringWheelAng[rad] : Demux  Outputs=[1]
  __TDD__LateralControl.SteeringWheelInputSwitch[-] : Demux  Outputs=[1]
  __TDD__LateralControl.SteeringWheelTrq[Nm] : Demux  Outputs=[1]
  __TDD__LateralControl.UserDefined1[-] : Demux  Outputs=[1]
  __TDD__LateralControl.UserDefined2[-] : Demux  Outputs=[1]
  __TDD__LateralControl.UserDefinedRefValue[-] : Demux  Outputs=[1]
  __TDO__LateralControl : BusCreator  Inputs=9
  LateralControl___UNIQUE_1 : Outport  Description=|  PortDimensions=[9]  VectorParamsAs1DForOutWhenUnconnected=off
      | <name>SteeringWheelAng[rad]</name>
      | <comment>Steering wheel angle</comment>
  wires:
  __TDO__LateralControl/1 -> LateralControl___UNIQUE_1/1  "LateralControl"
  __TDD__LateralControl.UserDefined2[-]/1 -> __TDO__LateralControl/9  "UserDefined2[-]"
  UserDefined2[-]___UNIQUE_1/1 -> __TDD__LateralControl.UserDefined2[-]/1  "UserDefined2[-]"
  __TDD__LateralControl.UserDefined1[-]/1 -> __TDO__LateralControl/8  "UserDefined1[-]"
  UserDefined1[-]___UNIQUE_1/1 -> __TDD__LateralControl.UserDefined1[-]/1  "UserDefined1[-]"
  __TDD__LateralControl.LateralPhase[-]/1 -> __TDO__LateralControl/7  "LateralPhase[-]"
  LateralPhase[-]___UNIQUE_1/1 -> __TDD__LateralControl.LateralPhase[-]/1  "LateralPhase[-]"
  __TDD__LateralControl.RightIndicator[0;1]/1 -> __TDO__LateralControl/6  "RightIndicator[0;1]"
  RightIndicator[0;1]___UNIQUE_1/1 -> __TDD__LateralControl.RightIndicator[0;1]/1  "RightIndicator[0;1]"
  __TDD__LateralControl.LeftIndicator[0;1]/1 -> __TDO__LateralControl/5  "LeftIndicator[0;1]"
  LeftIndicator[0;1]___UNIQUE_1/1 -> __TDD__LateralControl.LeftIndicator[0;1]/1  "LeftIndicator[0;1]"
  __TDD__LateralControl.UserDefinedRefValue[-]/1 -> __TDO__LateralControl/4  "UserDefinedRefValue[-]"
  UserDefinedRefValue[-]___UNIQUE_1/1 -> __TDD__LateralControl.UserDefinedRefValue[-]/1  "UserDefinedRefValue[-]"
  __TDD__LateralControl.SteeringWheelInputSwitch[-]/1 -> __TDO__LateralControl/3  "SteeringWheelInputSwitch[-]"
  SteeringWheelInputSwitch[-]___UNIQUE_1/1 -> __TDD__LateralControl.SteeringWheelInputSwitch[-]/1  "SteeringWheelInputSwitch[-]"
  __TDD__LateralControl.SteeringWheelTrq[Nm]/1 -> __TDO__LateralControl/2  "SteeringWheelTrq[Nm]"
  SteeringWheelTrq[Nm]___UNIQUE_1/1 -> __TDD__LateralControl.SteeringWheelTrq[Nm]/1  "SteeringWheelTrq[Nm]"
  __TDD__LateralControl.SteeringWheelAng[rad]/1 -> __TDO__LateralControl/1  "SteeringWheelAng[rad]"
  SteeringWheelAng[rad]___UNIQUE_1/1 -> __TDD__LateralControl.SteeringWheelAng[rad]/1  "SteeringWheelAng[rad]"

== system SingleTrack/VehicleControl/LateralControl/Enabled LateralControl/ControlSystems/SteeringWheelLimitation ==
  SteeringWheelDemands : Inport
  ControlInputs : Inport  Port=2
  Bus Selector1 : BusSelector  OutputSignals=MaxSteeringWheelRateLeft,MaxSteeringWheelRateRight,MaxSteeringWheelAngLeft,MaxSteeringWheelAngRight
  Bus Selector2 : BusSelector  OutputSignals=SteeringWheelAng[rad]
  LimitSteeringWheelAng : simulink/Discontinuities/Saturation Dynamic  OutMin=[]  OutMax=[]  OutDataTypeStr=Inherit: Same as second input  OutDataType=fixdt(1, 16)  OutScaling=2^-10  DoSatur=off
  LimitSteeringWheelGradient : simulink/Discontinuities/Rate Limiter Dynamic
      settings: SourceProductName=Simulink
  ModifiedSteeringWhlAng[rad] : Outport  VectorParamsAs1DForOutWhenUnconnected=off
  wires:
  Bus Selector2/1 -> LimitSteeringWheelGradient/2  "<SteeringWheelAng[rad]>"
  Bus Selector1/4 -> LimitSteeringWheelAng/3  "<MaxSteeringWheelAngRight>"
  Bus Selector1/3 -> LimitSteeringWheelAng/1  "<MaxSteeringWheelAngLeft>"
  Bus Selector1/2 -> LimitSteeringWheelGradient/3  "<MaxSteeringWheelRateRight>"
  Bus Selector1/1 -> LimitSteeringWheelGradient/1  "<MaxSteeringWheelRateLeft>"
  SteeringWheelDemands/1 -> Bus Selector2/1
  LimitSteeringWheelGradient/1 -> LimitSteeringWheelAng/2
  ControlInputs/1 -> Bus Selector1/1
  LimitSteeringWheelAng/1 -> ModifiedSteeringWhlAng[rad]/1  "SteeringWheelAng[rad]"

== system SingleTrack/VehicleControl/LateralControl/Enabled LateralControl/ControlSystemsPreprocessor/External Presetting of Controller  ==
  TaskIdentifiers : Inport
  SourceIdentifiers : Inport  Port=2
  ExtCtrlVariablesEnforced : Inport  Port=3
  Presetting Source Identifiers : Subsystem
  Presetting Task Identifiers : Subsystem
  ModifiedTaskIdentifiers : Outport  VectorParamsAs1DForOutWhenUnconnected=off
  ModifiedSourceIdentifiers : Outport  Port=2  VectorParamsAs1DForOutWhenUnconnected=off
  wires:
  Presetting Source Identifiers/1(ModifiedSourceIdentifiers) -> ModifiedSourceIdentifiers/1
  ExtCtrlVariablesEnforced/1 -> Presetting Task Identifiers/2("ExternalControlVariablesEnforced "), Presetting Source Identifiers/1("ExternalControlVariablesEnforced ")
  TaskIdentifiers/1 -> Presetting Task Identifiers/1(TaskIdentifiers)
  Presetting Task Identifiers/1(ModifiedTaskIdentifiers) -> ModifiedTaskIdentifiers/1
  SourceIdentifiers/1 -> Presetting Source Identifiers/2(SourceIdentifiers)

== system SingleTrack/VehicleControl/LateralControl/Enabled LateralControl/ControlSystemsPreprocessor/Generation of Guidance Data ==
  note: TASK_LAT_STEERING_WHEEL_ANG = 1;
      | 	TASK_LAT_STEERING_WHEEL_TORQUE = 2;
      | 	TASK_LAT_PATH_CONTROL = 3;
      | 	TASK_LAT_CURVATURE_CONTROL = 4;
      | 	TASK_LAT_USER_DEFINED = 5;
  TaskIdentifiers : Inport
  ControlInputs : Inport  Port=2
  ControllerParameters : Inport  Port=3
  VehicleInfo : Inport  Port=4
  Bus Creator : BusCreator  Inputs=20
  Bus Selector2 : BusSelector  OutputSignals=SteeringWheelAng,SteeringWheelTrq,RefLatPos,RefLane,RefPath,RefPathCurv,UserDefinedRefValue,LeftIndicator,RightIndicator,MaxSteeringWheelAngLeft,MaxSteeringWheelAngRight,MaxSteeringWheelRateLeft,MaxSteeringWheelRateRight
  Bus Selector6 : BusSelector  OutputSignals=Subtask,Task
  CurvatureGuidance : LateralControllerModules/CurvatureGuidance  sample_time=-1
  Demux : Demux  Outputs=7
  "Initialization, SteeringWheel, UserDefined" : Subsystem
  Merge : Merge  Inputs=3
  Mux : Mux  Inputs=2
  PathGuidance : LateralControllerModules/PathGuidance  sample_time=-1
  PreviousSubtask : Memory  InheritSampleTime=on
  Switch Case : SwitchCase  CaseConditions={vm_const('TASK_LAT_PATH_CONTROL'),vm_const('TASK_LAT_CURVATURE_CONTROL')}
  ExtendedControlInputs : Outport  VectorParamsAs1DForOutWhenUnconnected=off
  wires:
  [IRoadInterface] -> CurvatureGuidance/1, PathGuidance/1
  Bus Selector2/13 -> Bus Creator/20  "<MaxSteeringWheelRateRight>"
  Bus Selector2/12 -> Bus Creator/19  "<MaxSteeringWheelRateLeft>"
  Bus Selector2/2 -> Bus Creator/9  "<SteeringWheelTrq>"
  Bus Selector2/3 -> Bus Creator/10  "<RefLatPos>"
  Bus Selector2/11 -> Bus Creator/18  "<MaxSteeringWheelAngRight>"
  Bus Selector2/10 -> Bus Creator/17  "<MaxSteeringWheelAngLeft>"
  Bus Selector2/4 -> Bus Creator/11  "<RefLane>"
  Bus Selector2/9 -> Bus Creator/16  "<RightIndicator>"
  Bus Selector2/5 -> Bus Creator/12  "<RefPath>"
  Bus Selector2/8 -> Bus Creator/15  "<LeftIndicator>"
  Bus Selector2/6 -> Bus Creator/13  "<RefPathCurv>"
  Bus Selector2/7 -> Bus Creator/14  "<UserDefinedRefValue>"
  "Initialization, SteeringWheel, UserDefined"/1(TargetAndTargetAim) -> Merge/3
  PreviousSubtask/1 -> Mux/2
  Mux/1 -> PathGuidance/2, CurvatureGuidance/2
  Merge/1 -> Demux/1
  CurvatureGuidance/1 -> Merge/2
  PathGuidance/1 -> Merge/1
  Bus Creator/1 -> ExtendedControlInputs/1
  Switch Case/3 -> "Initialization, SteeringWheel, UserDefined"/Action
  Switch Case/2 -> CurvatureGuidance/Action
  Switch Case/1 -> PathGuidance/Action
  Bus Selector6/1 -> PreviousSubtask/1, Mux/1  "<Subtask>"
  Bus Selector6/2 -> Switch Case/1  "<Task>"
  TaskIdentifiers/1 -> Bus Selector6/1
  ControllerParameters/1 -> CurvatureGuidance/4, PathGuidance/4
  VehicleInfo/1 -> PathGuidance/5, CurvatureGuidance/5
  ControlInputs/1 -> CurvatureGuidance/3, Bus Selector2/1, PathGuidance/3
  Bus Selector2/1 -> Bus Creator/8  "<SteeringWheelAng>"
  Demux/1 -> Bus Creator/1  "tgt_x"
  Demux/2 -> Bus Creator/2  "tgt_y"
  Demux/3 -> Bus Creator/3  "tgt_z"
  Demux/4 -> Bus Creator/4  "tgt_cu"
  Demux/5 -> Bus Creator/5  "tgt_psi"
  Demux/6 -> Bus Creator/6  "taim_x"
  Demux/7 -> Bus Creator/7  "taim_y"

== system SingleTrack/VehicleControl/LateralControl/Enabled LateralControl/ControlSystemsPreprocessor/Generation of Hold Data ==
  PhaseTrigger : Inport
  LatCTRL : Inport  Port=2
  VehicleInfo : Inport  Port=3
  Bus Selector18 : BusSelector  OutputSignals=VehicleRoadInfo_RoadQ[m],VehicleRoadInfo_LaneID[-],VehicleRoadInfo_LaneCurvature[1/m]  OutputAsBus=on
  Enabled Subsystem : Subsystem  TreatAsAtomicUnit=on
  Memory : Memory  InheritSampleTime=on
  Memory1 : Memory  InheritSampleTime=on
  HoldData : Outport  VectorParamsAs1DForOutWhenUnconnected=off
  wires:
  Memory1/1 -> Enabled Subsystem/2(VehicleInfo)
  Memory/1 -> Enabled Subsystem/1(LatCTRL)
  Bus Selector18/1 -> Memory1/1
  VehicleInfo/1 -> Bus Selector18/1
  Enabled Subsystem/1(HoldData) -> HoldData/1
  LatCTRL/1 -> Memory/1
  PhaseTrigger/1 -> Enabled Subsystem/Enable

== system SingleTrack/VehicleControl/LateralControl/Enabled LateralControl/ControlSystemsPreprocessor/Switch between Data Sources ==
  note: SOURCE_NOMINALPATH = 1;
      | 	SOURCE_LANE = 2;
      | 	SOURCE_CONSTANT = 3;
      | 	SOURCE_TABLE_DISCRETE = 4;
      | 	SOURCE_TABLE_LINEAR = 5;
      | 	SOURCE_TABLE_CUBIC = 6;
      | 	SOURCE_TABLE_HAVERSINE = 7;
      | 	SOURCE_AUTOMATIC = 8;
      | 	SOURCE_SINE_TIME = 9;
      | 	SOURCE_SINE_PATH = 10;
      | 	SOURCE_HOLD = 11;
      | 	SOURCE_EXTERNAL = 12;
      | 	SOURCE_EXTERNAL_NOMINALPATH = 13;
      | 	SOURCE_EXTERNAL_LANE = 14;
  SourceIdentifiers : Inport
  ControlInputs : Inport  Port=2  OutDataTypeStr=Bus: TD_BO_LateralControlInputs
  HoldData : Inport  Port=3  OutDataTypeStr=Bus: TD_BO_LateralControlInputs
  ExternalData : Inport  Port=4  OutDataTypeStr=Bus: TD_BO_LateralControlInputs
  Add : Sum  Inputs=3  AccumDataTypeStr=uint8
  Bus to Vector{,1..3} (4 alike) : BusToVector
  Constant : Constant
  LateralControlDefaultInputs_Vector2Object : LateralControllerModules/LateralControlDefaultInputs_Vector2Object  SystemSampleTime=-1  Latency=0  AutoFrameSizeCalculation=off
  MinMax : MinMax  Inputs=2  OutDataTypeStr=uint8
  Multiport Switch Zero Based : MultiPortSwitch  DataPortForDefault=Additional data port  DiagnosticForDefault=None
  NonVirtualToVirtual1 : SignalConversion  ConversionOutput=Virtual bus  OverrideOpt=off
  NonVirtualToVirtual2 : SignalConversion  ConversionOutput=Virtual bus  OverrideOpt=off
  defaultValue : Constant  Value=zeros(1,vm_const('NUM_SIGNALS_LATERALMANEUVER'))
  isExternal : simulink/Logic and Bit Operations/Compare To Constant  relop=>=  const=vm_const('SOURCE_EXTERNAL')  OutDataTypeStr=uint8  ZeroCross=off
  isHold : simulink/Logic and Bit Operations/Compare To Constant  relop=>=  const=vm_const('SOURCE_HOLD')  OutDataTypeStr=uint8  ZeroCross=off
  SwitchedControlInputs : Outport  VectorParamsAs1DForOutWhenUnconnected=off
  wires:
  Add/1 -> Multiport Switch Zero Based/1
  NonVirtualToVirtual2/1 -> Bus to Vector3/1
  NonVirtualToVirtual1/1 -> Bus to Vector2/1
  Bus to Vector3/1 -> Multiport Switch Zero Based/4
  Bus to Vector2/1 -> Multiport Switch Zero Based/3
  defaultValue/1 -> Multiport Switch Zero Based/5
  Constant/1 -> MinMax/1
  ExternalData/1 -> NonVirtualToVirtual2/1
  Bus to Vector1/1 -> Multiport Switch Zero Based/2
  MinMax/1 -> Add/1
  Bus to Vector/1 -> isHold/1, MinMax/2, isExternal/1
  isExternal/1 -> Add/3
  isHold/1 -> Add/2
  LateralControlDefaultInputs_Vector2Object/1 -> SwitchedControlInputs/1
  Multiport Switch Zero Based/1 -> LateralControlDefaultInputs_Vector2Object/1
  HoldData/1 -> NonVirtualToVirtual1/1
  ControlInputs/1 -> Bus to Vector1/1
  SourceIdentifiers/1 -> Bus to Vector/1

== system SingleTrack/VehicleControl/LongitudinalControl/ControlSystems/Brake System Switch and Pedal Limitation/AccBrakeLimitation ==
  AccPedalPos[0_1] : Inport
  BrakePedalPos[0_1] : Inport  Port=2
  ControlInputs : Inport  Port=3
  BusSelector : BusSelector  OutputSignals=MaxAccPedalCloseSlewRate,MaxAccPedalOpenSlewRate,MaxBrakePedalCloseSlewRate,MaxBrakePedalOpenSlewRate,MaxAccPedalPos,MaxBrakePedalPos
  Constant : Constant  Value=0
  Constant1 : Constant  Value=0
  LimitAccPedalGradient : simulink/Discontinuities/Rate Limiter Dynamic
      settings: SourceProductName=Simulink
  LimitAccPedalPos : simulink/Discontinuities/Saturation Dynamic  OutMin=[]  OutMax=[]  OutDataTypeStr=Inherit: Same as second input  OutDataType=fixdt(1, 16)  OutScaling=2^-10  DoSatur=off
  LimitBrakePedalGradient : simulink/Discontinuities/Rate Limiter Dynamic
      settings: SourceProductName=Simulink
  LimitBrakePedalPos : simulink/Discontinuities/Saturation Dynamic  OutMin=[]  OutMax=[]  OutDataTypeStr=Inherit: Same as second input  OutDataType=fixdt(1, 16)  OutScaling=2^-10  DoSatur=off
  AccPedalPosLimited : Outport  VectorParamsAs1DForOutWhenUnconnected=off
  BrakePedalPosLimited : Outport  Port=2  VectorParamsAs1DForOutWhenUnconnected=off
  wires:
  LimitAccPedalPos/1 -> AccPedalPosLimited/1
  LimitBrakePedalPos/1 -> BrakePedalPosLimited/1
  BrakePedalPos[0_1]/1 -> LimitBrakePedalGradient/2
  ControlInputs/1 -> BusSelector/1
  BusSelector/5 -> LimitAccPedalPos/1  "<MaxAccPedalPos>"
  BusSelector/6 -> LimitBrakePedalPos/1  "<MaxBrakePedalPos>"
  LimitAccPedalGradient/1 -> LimitAccPedalPos/2
  LimitBrakePedalGradient/1 -> LimitBrakePedalPos/2
  Constant/1 -> LimitAccPedalPos/3
  Constant1/1 -> LimitBrakePedalPos/3
  BusSelector/1 -> LimitAccPedalGradient/1  "<MaxAccPedalCloseSlewRate>"
  BusSelector/2 -> LimitAccPedalGradient/3  "<MaxAccPedalOpenSlewRate>"
  BusSelector/3 -> LimitBrakePedalGradient/1  "<MaxBrakePedalCloseSlewRate>"
  BusSelector/4 -> LimitBrakePedalGradient/3  "<MaxBrakePedalOpenSlewRate>"
  AccPedalPos[0_1]/1 -> LimitAccPedalGradient/2

== system SingleTrack/VehicleControl/LongitudinalControl/ControlSystems/Brake System Switch and Pedal Limitation/BrakeSwitch = 1 ==
  BrakePedalPos : Inport
  WheelBrakePressures : Inport  Port=2
  Action Port : ActionPort  InitializeStates=reset  PropagateVarSize=During execution  ActionPortLabel=case [ 1 ]:
  Bus Creator : BusCreator  Inputs=2
  Bus to Vector : BusToVector
  MinMax : MinMax  Function=max
  BrakeOutput : Outport  VectorParamsAs1DForOutWhenUnconnected=off
  wires:
  Bus to Vector/1 -> MinMax/1
  WheelBrakePressures/1 -> Bus to Vector/1
  MinMax/1 -> Bus Creator/2  "MainBrakePressure"
  BrakePedalPos/1 -> Bus Creator/1  "BrakePedalPos"
  Bus Creator/1 -> BrakeOutput/1

== system SingleTrack/VehicleControl/LongitudinalControl/ControlSystems/Brake System Switch and Pedal Limitation/BrakeSwitch = 2 ==
  MainBrakePressure : Inport
  MaxMainBrakePressure : Inport  Port=2
  Action Port : ActionPort  InitializeStates=reset  PropagateVarSize=During execution  ActionPortLabel=case [ 2 ]:
  Bus Creator : BusCreator  Inputs=2
  Divide : Product  Inputs=/*
  Saturation : Saturate  UpperLimit=inf  LowerLimit=1e-6
  Signal Conversion : SignalConversion  OverrideOpt=off
  BrakeOutput : Outport  VectorParamsAs1DForOutWhenUnconnected=off
  wires:
  Saturation/1 -> Divide/1
  MainBrakePressure/1 -> Bus Creator/2, Divide/2  "MainBrakePressure"
  Divide/1 -> Bus Creator/1  "BrakePedalPos"
  Bus Creator/1 -> Signal Conversion/1
  Signal Conversion/1 -> BrakeOutput/1
  MaxMainBrakePressure/1 -> Saturation/1

== system SingleTrack/VehicleControl/LongitudinalControl/ControlSystems/Brake System Switch and Pedal Limitation/Default ==
  WheelBrakePressures : Inport
  MaxMainBrakePressure : Inport  Port=2
  Action Port : ActionPort  InitializeStates=reset  PropagateVarSize=During execution  ActionPortLabel=default:
  Bus Creator : BusCreator  Inputs=2
  Bus to Vector : BusToVector
  Divide : Product  Inputs=/*
  MinMax : MinMax  Function=max
  Saturation : Saturate  UpperLimit=inf  LowerLimit=1e-6
  Signal Conversion : SignalConversion  OverrideOpt=off
  BrakeOutput : Outport  VectorParamsAs1DForOutWhenUnconnected=off
  wires:
  Saturation/1 -> Divide/1
  WheelBrakePressures/1 -> Bus to Vector/1
  Divide/1 -> Bus Creator/1  "BrakePedalPos"
  Bus to Vector/1 -> MinMax/1
  MinMax/1 -> Bus Creator/2, Divide/2  "MainBrakePressure"
  Bus Creator/1 -> Signal Conversion/1
  Signal Conversion/1 -> BrakeOutput/1
  MaxMainBrakePressure/1 -> Saturation/1
